simulink model "zumo_PID_controller_raw_values"  (R2014b)
settings: Solver=ode3  SolverMode=SingleTasking  StartTime=0.0  StopTime=4  FixedStep=0.01  RelTol=1e-3
InitFcn:
  | mapdata = processmap('mapTrackA.mat');
model workspace (MAT data in the model file):
  axleLength = Simulink.Parameter
  axleLength.Value = 9.8
  axleLength.Description = 'Distance between tire contact points
    | of the two wheels/treads
    | in units of centimeters.'
  axleLength.DataType = 'auto'
  commandPercmPerSecond = Simulink.Parameter
  commandPercmPerSecond.Value = 3.9547
  commandPercmPerSecond.Description = 'Convert units of ''command'' 
    | to units of ''cm/s''.
    | 
    | ''command'' is a value in the range [-256, 255].'
  commandPercmPerSecond.DataType = 'auto'
  symmetrizeMotors = Simulink.Parameter
  symmetrizeMotors.Value = 1
  symmetrizeMotors.Description = 'Scale one of the motor commands down 
    | (not up) to balance the motors. 
    | Once balanced, a value of x sent to either
    | motor will produce the same rate of rotation
    | in both motors.'
  symmetrizeMotors.DataType = 'auto'
  sampleTime = Simulink.Parameter
  sampleTime.Value = 0.01
  sampleTime.Description = 'Sample time (in seconds) of the trajectory simulator.'
  sampleTime.DataType = 'auto'
  commandThreshold = Simulink.Parameter
  commandThreshold.Value = 31.875
  commandThreshold.DataType = 'auto'
  lineThreshold = Simulink.Parameter
  lineThreshold.Value = 900
  lineThreshold.DataType = 'auto'
  velocity = Simulink.Parameter
  velocity.Value = 15
  velocity.Description = 'cm / s'
  velocity.DataType = 'auto'
  waveLength = Simulink.Parameter
  waveLength.Value = 8.6
  waveLength.Description = 'Units of cm.
    | 
    | The following condition must be satisfied: 
    | waveLength > 2*pi * velocity / sqrt(0.5 / sampleTime)
    | 
    | For reference,
    | robotLength = 8.6 cm
    | '
  waveLength.DataType = 'auto'
libraries: simulink x2, ZumoBotLib x2, arduinolib x1
settings Model: ExtModeTrigDuration=2  Creator=pkasseba  LastModifiedBy=sandip
settings OptimizationCC: OptimizeModelRefInitCode=on  LifeSpan=1
settings DebuggingCC: UnderspecifiedInitializationDetection=Classic  MergeDetectMultiDrivingBlocksExec=none  SolverPrmCheckMsg=none  StateNameClashWarn=warning
settings HardwareCC: ProdBitPerInt=16  ProdBitPerPointer=8  ProdIntDivRoundTo=Zero  ProdEndianess=LittleEndian  ProdWordSize=8  ProdHWDeviceType=Atmel->AVR
settings SFSimCC: SimParseCustomCode=off
settings RTWCC: SystemTargetFile=realtime.tlc  GenerateMakefile=off  TemplateMakefile=realtime.tmf  Description=Run on Target Hardware  RTWVerbose=off  ProcessScript=realtime_make_rtw_hook
settings STFCustomTargetCC: TargetLibSuffix=.a  GenerateSampleERTMain=on  ERTCustomFileBanners=on  SupportNonInlinedSFcns=off  SupportVariableSizeSignals=on  MATLABClassNameForMDSCustomization=Simulink.SoftwareTarget.ERTCustomization  GRTInterface=off  SystemTargetFile=realtime.tlc
settings ERTTargetCC: GenerateSampleERTMain=on  ParMdlRefBuildCompliant=off  CompOptLevelCompliant=off  ConcurrentExecutionCompliant=off  CombineOutputUpdateFcns=off  ERTFirstTimeCompliant=off  SupportContinuousTime=on  SupportVariableSizeSignals=on  ModelStepFunctionPrototypeControlCompliant=off  CPPClassGenCompliant=off  ExtModeTransport=3  ExtModeMexFile=ext_serial_win32_comm  ExtModeMexArgs=0 1 9600  InlinedParameterPlacement=NonHierarchical  ERTSrcFileBannerTemplate=realtime_code_template.cgt  ERTHdrFileBannerTemplate=realtime_code_template.cgt  ERTDataSrcFileTemplate=realtime_code_template.cgt  ERTDataHdrFileTemplate=realtime_code_template.cgt  ERTCustomFileTemplate=realtime_file_process.tlc

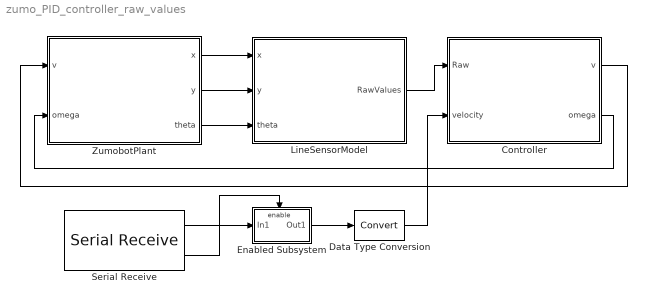
== system zumo_PID_controller_raw_values ==
  Controller : Subsystem
  Data Type Conversion : DataTypeConversion
  Enabled Subsystem : Subsystem  TreatAsAtomicUnit=on
  LineSensorModel : Subsystem  Variant=on
  Serial Receive : arduinolib/Serial Receive  portNumber=0  showOutStatus=on  sampleTime=0.02  blockPlatform=arduino
  ZumobotPlant : Subsystem  Variant=on
  wires:
  Controller/1(v) -> ZumobotPlant/1(v)
  ZumobotPlant/1(x) -> LineSensorModel/1(x)
  ZumobotPlant/2(y) -> LineSensorModel/2(y)
  LineSensorModel/1(RawValues) -> Controller/1(Raw)
  Controller/2(omega) -> ZumobotPlant/2(omega)
  ZumobotPlant/3(theta) -> LineSensorModel/3(theta)
  Serial Receive/1 -> Enabled Subsystem/1(In1)
  Serial Receive/2 -> Enabled Subsystem/Enable
  Enabled Subsystem/1(Out1) -> Data Type Conversion/1
  Data Type Conversion/1 -> Controller/2(velocity)

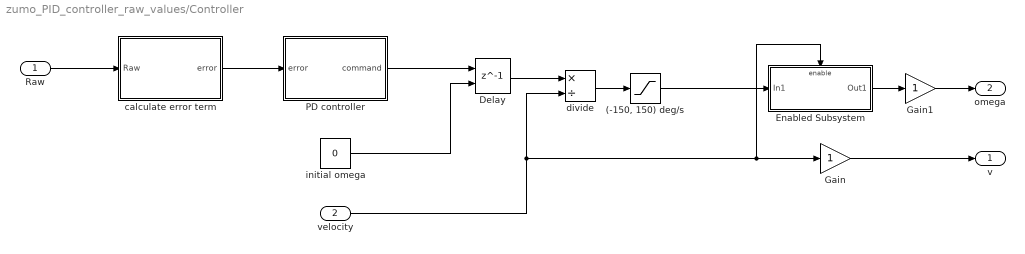
== system zumo_PID_controller_raw_values/Controller ==
  Raw : Inport
  velocity : Inport  Port=2
  "(-150, 150) deg/s" : Saturate  UpperLimit=150*pi/180  LowerLimit=-150*pi/180
  Delay : Delay  DelayLength=1  InitialConditionSource=Input port  InitialCondition=0
      settings: InputPortMap=u0,p4
  Enabled Subsystem : Subsystem  TreatAsAtomicUnit=on
  Gain : Gain
  Gain1 : Gain
  PD controller : Subsystem
  calculate error term : Subsystem
  divide : Product  Inputs=*/
  initial omega : Constant  Value=0
  v : Outport
  omega : Outport  Port=2
  wires:
  velocity/1 -> Gain/1, Enabled Subsystem/Enable, divide/2
  Delay/1 -> divide/1
  initial omega/1 -> Delay/2
  Raw/1 -> calculate error term/1(Raw)
  divide/1 -> "(-150, 150) deg/s"/1
  calculate error term/1(error) -> PD controller/1(error)
  PD controller/1(command) -> Delay/1
  "(-150, 150) deg/s"/1 -> Enabled Subsystem/1(In1)
  Enabled Subsystem/1(Out1) -> Gain1/1
  Gain/1 -> v/1
  Gain1/1 -> omega/1

== system zumo_PID_controller_raw_values/Enabled Subsystem ==
  In1 : Inport
  Enable : EnablePort
  Out1 : Outport  InitialOutput=0
  wires:
  In1/1 -> Out1/1

== system zumo_PID_controller_raw_values/LineSensorModel ==
  note: 1) Only subsystems can be added as variant choices at this level
      | 2) Blocks cannot be connected at this level as connectivity is
      | automatically determined at simulation, based on the active variant
  x : Inport
  y : Inport  Port=2
  theta : Inport  Port=3
  Simulation : Subsystem  VariantControl=sim==1
  Target : Subsystem  VariantControl=sim==0
  RawValues : Outport

== system zumo_PID_controller_raw_values/ZumobotPlant ==
  note: 1) Only subsystems can be added as variant choices at this level
      | 2) Blocks cannot be connected at this level as connectivity is
      | automatically determined at simulation, based on the active variant
  v : Inport
  omega : Inport  Port=2
  Simulation : Subsystem  VariantControl=sim==1
  Target : Subsystem  VariantControl=sim==0
  x : Outport
  y : Outport  Port=2
  theta : Outport  Port=3

== system zumo_PID_controller_raw_values/Controller/Enabled Subsystem ==
  In1 : Inport
  Enable : EnablePort
  Out1 : Outport  OutputWhenDisabled=reset  InitialOutput=0
  wires:
  In1/1 -> Out1/1

== system zumo_PID_controller_raw_values/Controller/PD controller ==
  error : Inport
  2*alpha : Gain  Gain=2*(2*pi*velocity/waveLength)
  Discrete Derivative : simulink/Discrete/Discrete Derivative  gainval=1.0  ICPrevScaledInput=0.0  InputProcessing=Inherited  OutMin=[]  OutMax=[]  OutDataType=fixdt(1, 16)  OutScaling=2^-10  DoSatur=off
  Sum : Sum  Inputs=|++
  alpha^2 : Gain  Gain=(2*pi*velocity/waveLength)^2
  zeta : Gain  Gain=0.4
  command : Outport
  wires:
  zeta/1 -> 2*alpha/1
  2*alpha/1 -> Discrete Derivative/1
  alpha^2/1 -> Sum/1
  Sum/1 -> command/1
  Discrete Derivative/1 -> Sum/2
  error/1 -> alpha^2/1, zeta/1

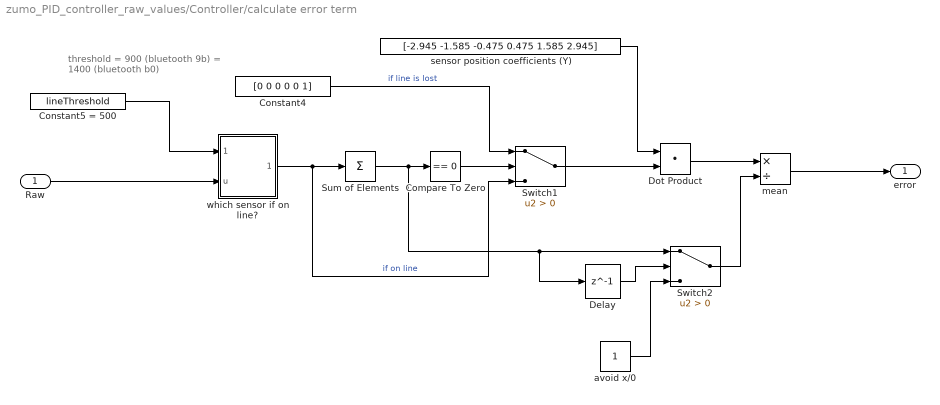
== system zumo_PID_controller_raw_values/Controller/calculate error term ==
  note: threshold = 900 (bluetooth 9b)
      | = 1400 (bluetooth b0)
  Raw : Inport
  Compare To Zero : simulink/Logic and Bit Operations/Compare To Zero  relop===  OutDataTypeStr=boolean
  Constant4 : Constant  Value=[0 0 0 0 0 1]
  Constant5 = 500 : Constant  Value=lineThreshold
  Delay : Delay  DelayLength=1  InitialCondition=0
  Dot Product : DotProduct  InputSameDT=on  OutDataTypeStr=Inherit: Inherit via internal rule
  Sum of Elements : Sum  Inputs=+
  Switch1 : Switch  Criteria=u2 > Threshold
  Switch2 : Switch  Criteria=u2 > Threshold
  avoid x/0 : Constant
  mean : Product  Inputs=*/
  sensor position coefficients (Y) : Constant  Value=[-2.945 -1.585 -0.475 0.475 1.585 2.945]
  which sensor if on line? : Subsystem
  error : Outport
  wires:
  Constant4/1 -> Switch1/1  "if line is lost"
  Constant5 = 500/1 -> which sensor if on line?/1(threshold)
  Dot Product/1 -> mean/1
  sensor position coefficients (Y)/1 -> Dot Product/1
  Raw/1 -> which sensor if on line?/2(u)
  which sensor if on line?/1(Out1) -> Switch1/3, Sum of Elements/1  "if on line"
  Switch2/1 -> mean/2
  avoid x/0/1 -> Switch2/3
  Switch1/1 -> Dot Product/2
  mean/1 -> error/1
  Compare To Zero/1 -> Switch1/2
  Sum of Elements/1 -> Delay/1, Switch2/1, Compare To Zero/1
  Delay/1 -> Switch2/2

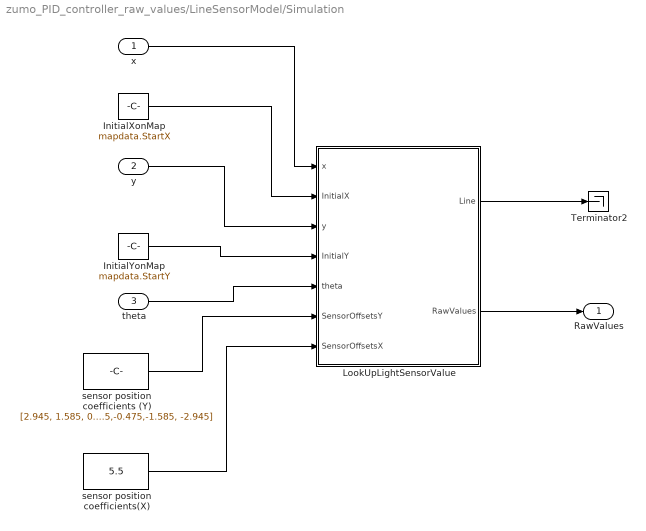
== system zumo_PID_controller_raw_values/LineSensorModel/Simulation ==
  x : Inport
  y : Inport  Port=2
  theta : Inport  Port=3
  InitialXonMap : Constant  Value=mapdata.StartX
  InitialYonMap : Constant  Value=mapdata.StartY
  LookUpLightSensorValue : Subsystem
  Terminator2 : Terminator
  sensor position coefficients (Y) : Constant  Value=[2.945, 1.585, 0.475,-0.475,-1.585, -2.945]
  sensor position coefficients(X) : Constant  Value=5.5
  RawValues : Outport
  wires:
  LookUpLightSensorValue/1(Line) -> Terminator2/1
  LookUpLightSensorValue/2(RawValues) -> RawValues/1
  InitialYonMap/1 -> LookUpLightSensorValue/4(InitialY)
  theta/1 -> LookUpLightSensorValue/5(theta)
  sensor position coefficients (Y)/1 -> LookUpLightSensorValue/6(SensorOffsetsY)
  y/1 -> LookUpLightSensorValue/3(y)
  InitialXonMap/1 -> LookUpLightSensorValue/2(InitialX)
  x/1 -> LookUpLightSensorValue/1(x)
  sensor position coefficients(X)/1 -> LookUpLightSensorValue/7(SensorOffsetsX)

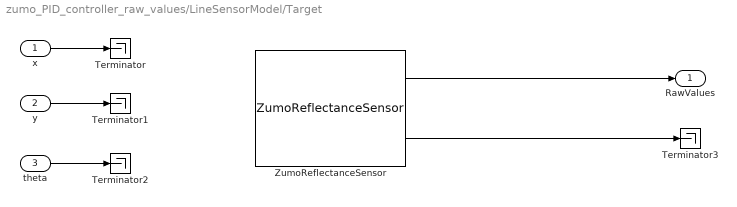
== system zumo_PID_controller_raw_values/LineSensorModel/Target ==
  x : Inport
  y : Inport  Port=2
  theta : Inport  Port=3
  Terminator{,1..3} (4 alike) : Terminator
  ZumoReflectanceSensor : ZumoBotLib/ZumoReflectanceSensor  sampleTime_dd=0.02  emitterPin_dd=255  debug_dd=off
  RawValues : Outport
  wires:
  ZumoReflectanceSensor/1 -> RawValues/1
  ZumoReflectanceSensor/2 -> Terminator3/1
  x/1 -> Terminator/1
  y/1 -> Terminator1/1
  theta/1 -> Terminator2/1

== system zumo_PID_controller_raw_values/ZumobotPlant/Simulation ==
  v : Inport
  omega : Inport  Port=2
  motor command conversion : Subsystem
  simulated trajectory : Subsystem
  x : Outport
  y : Outport  Port=2
  theta : Outport  Port=3
  wires:
  v/1 -> motor command conversion/1(v)
  simulated trajectory/1(x) -> x/1
  simulated trajectory/2(y) -> y/1
  motor command conversion/1(v_L v_R) -> simulated trajectory/1(v_L v_R)
  omega/1 -> motor command conversion/2(omega)
  simulated trajectory/3(theta) -> theta/1

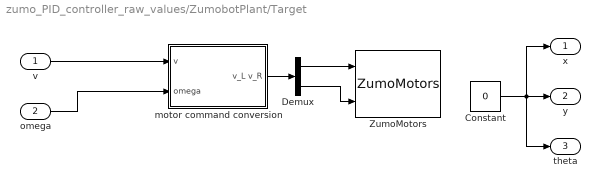
== system zumo_PID_controller_raw_values/ZumobotPlant/Target ==
  v : Inport
  omega : Inport  Port=2
  Constant : Constant  Value=0
  Demux : Demux  Outputs=2
  ZumoMotors : ZumoBotLib/ZumoMotors  flipLeft=off  flipRight=off
  motor command conversion : Subsystem
  x : Outport
  y : Outport  Port=2
  theta : Outport  Port=3
  wires:
  motor command conversion/1(v_L v_R) -> Demux/1
  Demux/1 -> ZumoMotors/1
  Demux/2 -> ZumoMotors/2
  v/1 -> motor command conversion/1(v)
  omega/1 -> motor command conversion/2(omega)
  Constant/1 -> theta/1, x/1, y/1

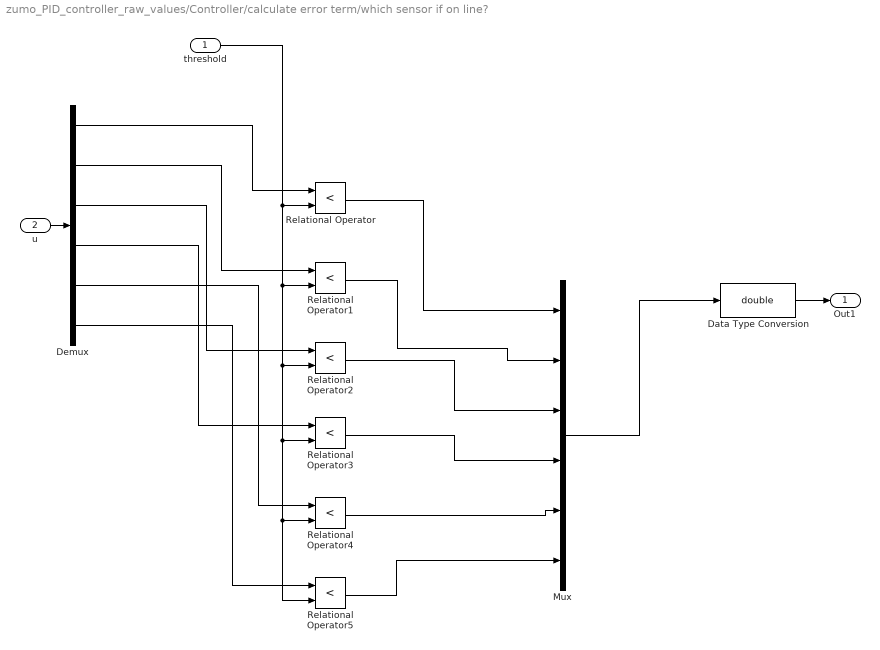
== system zumo_PID_controller_raw_values/Controller/calculate error term/which sensor if on line? ==
  threshold : Inport
  u : Inport  Port=2
  Data Type Conversion : DataTypeConversion  OutDataTypeStr=double
  Demux : Demux  Outputs=6
  Mux : Mux  Inputs=6
  Relational Operator{,1..5} (6 alike) : RelationalOperator  Operator=<  OutDataTypeStr=boolean
  Out1 : Outport
  wires:
  Mux/1 -> Data Type Conversion/1
  u/1 -> Demux/1
  Demux/1 -> Relational Operator/1
  Demux/2 -> Relational Operator1/1
  Demux/3 -> Relational Operator2/1
  Demux/4 -> Relational Operator3/1
  Demux/5 -> Relational Operator4/1
  Demux/6 -> Relational Operator5/1
  threshold/1 -> Relational Operator5/2, Relational Operator4/2, Relational Operator3/2, Relational Operator2/2, Relational Operator1/2, Relational Operator/2
  Relational Operator1/1 -> Mux/2
  Relational Operator2/1 -> Mux/3
  Relational Operator/1 -> Mux/1
  Relational Operator3/1 -> Mux/4
  Relational Operator5/1 -> Mux/6
  Data Type Conversion/1 -> Out1/1
  Relational Operator4/1 -> Mux/5

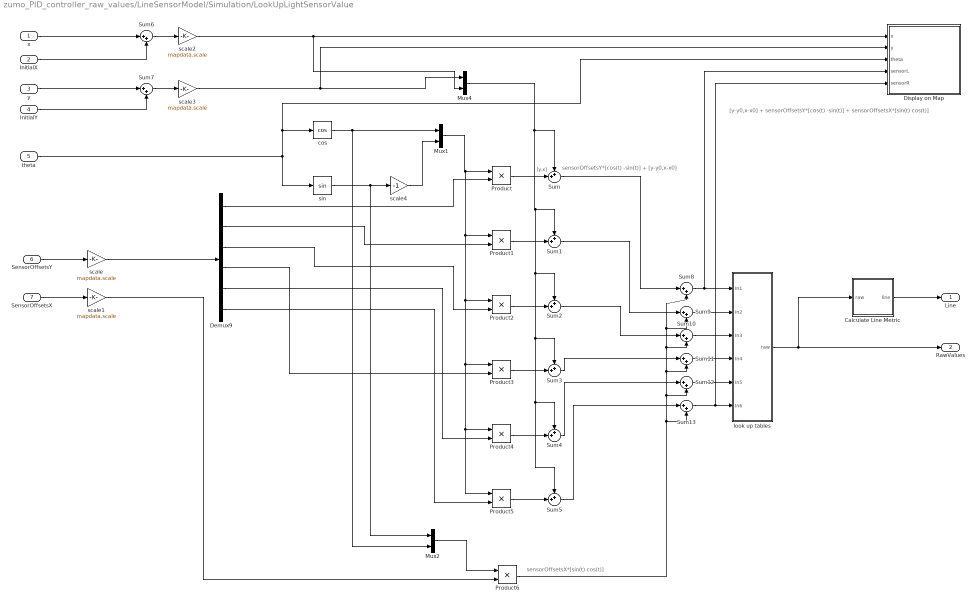
== system zumo_PID_controller_raw_values/LineSensorModel/Simulation/LookUpLightSensorValue ==
  note: [y-y0,x-x0] + sensorOffsetsY*[cos(t) -sin(t)] + sensorOffsetsX*[sin(t) cos(t)]
  note: sensorOffsetsY*[cos(t) -sin(t)] + [y-y0,x-x0]
  note: sensorOffsetsX*[sin(t) cos(t)]
  x : Inport
  InitialX : Inport  Port=2
  y : Inport  Port=3
  InitialY : Inport  Port=4
  theta : Inport  Port=5
  SensorOffsetsY : Inport  Port=6
  SensorOffsetsX : Inport  Port=7
  Calculate Line Metric : Subsystem
  Demux9 : Demux  Outputs=6
  Display on Map : MATLAB Function  TreatAsAtomicUnit=on
  Mux1 : Mux  Inputs=2
  Mux2 : Mux  Inputs=2
  Mux4 : Mux  Inputs=2
  Product{,1..6} (7 alike) : Product
  Sum{,1..5} (6 alike) : Sum  Inputs=++|
  Sum{6..13} (8 alike) : Sum  Inputs=|++
  cos : Trigonometry  Operator=cos
  look up tables : Subsystem
  scale{,1..3} (4 alike) : Gain  Gain=mapdata.scale
  scale4 : Gain  Gain=-1
  sin : Trigonometry
  Line : Outport
  RawValues : Outport  Port=2
  wires:
  SensorOffsetsY/1 -> scale/1
  Mux1/1 -> Product5/1, Product4/1, Product3/1, Product2/1, Product1/1, Product/1
  Product/1 -> Sum/2
  Product1/1 -> Sum1/2
  Product2/1 -> Sum2/2
  Product4/1 -> Sum4/2
  Product3/1 -> Sum3/2
  Product5/1 -> Sum5/2
  Sum/1 -> Sum8/1
  Sum5/1 -> Sum13/1
  scale/1 -> Demux9/1
  Demux9/4 -> Product3/2
  Demux9/5 -> Product4/2
  Demux9/3 -> Product2/2
  Demux9/6 -> Product5/2
  Demux9/2 -> Product1/2
  Demux9/1 -> Product/2
  Mux4/1 -> Sum/1, Sum5/1, Sum4/1, Sum3/1, Sum2/1, Sum1/1  "[y,x]"
  SensorOffsetsX/1 -> scale1/1
  scale1/1 -> Product6/2
  Mux2/1 -> Product6/1
  Product6/1 -> Sum13/2, Sum12/2, Sum11/2, Sum10/2, Sum9/2, Sum8/2
  x/1 -> Sum6/1
  Sum6/1 -> scale2/1
  InitialX/1 -> Sum6/2
  y/1 -> Sum7/1
  Sum7/1 -> scale3/1
  InitialY/1 -> Sum7/2
  scale2/1 -> Mux4/2, Display on Map/1(x)
  scale3/1 -> Mux4/1, Display on Map/2(y)
  Calculate Line Metric/1(line) -> Line/1
  look up tables/1(raw) -> Calculate Line Metric/1(raw), RawValues/1
  Sum1/1 -> Sum9/1
  Sum2/1 -> Sum10/1
  Sum3/1 -> Sum11/1
  Sum4/1 -> Sum12/1
  Sum8/1 -> Display on Map/4(sensorL), look up tables/1(In1)
  Sum9/1 -> look up tables/2(In2)
  Sum10/1 -> look up tables/3(In3)
  Sum11/1 -> look up tables/4(In4)
  Sum12/1 -> look up tables/5(In5)
  Sum13/1 -> Display on Map/5(sensorR), look up tables/6(In6)
  sin/1 -> Mux2/1, scale4/1
  cos/1 -> Mux2/2, Mux1/1
  theta/1 -> Display on Map/3(theta), cos/1, sin/1
  scale4/1 -> Mux1/2

== system zumo_PID_controller_raw_values/ZumobotPlant/Simulation/motor command conversion ==
  note: or in matrix notation,
  note: v_L  = v - omega * axleLength/2
      | v_R = v + omega * axleLength/2
  note: [v_L; v_R] = [1 -axleLength/2; 1 axleLength/2] * [v; omega]
  v : Inport
  omega : Inport  Port=2
  Mux : Mux  Inputs=2
  Saturation [-256 255] : Saturate  UpperLimit=255  LowerLimit=-256
  change parameters : Gain  Gain=[1 -axleLength/2; 1 axleLength/2]  Multiplication=Matrix(K*u)
  change units : Gain  Gain=commandPercmPerSecond
  symmetrize motors : Gain  Gain=[1 symmetrizeMotors]
  v_L v_R : Outport
  wires:
  change parameters/1 -> symmetrize motors/1  "v_L v_R"
  change units/1 -> Saturation [-256 255]/1  "v_L v_R (command)"
  symmetrize motors/1 -> change units/1  "v_L v_R (cm/s)"
  Saturation [-256 255]/1 -> v_L v_R/1
  Mux/1 -> change parameters/1
  omega/1 -> Mux/2
  v/1 -> Mux/1

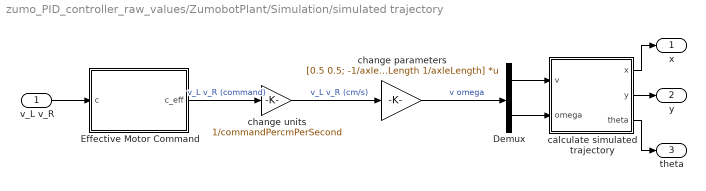
== system zumo_PID_controller_raw_values/ZumobotPlant/Simulation/simulated trajectory ==
  v_L v_R : Inport
  Demux : Demux  Outputs=2
  Effective Motor Command : Subsystem
  calculate simulated trajectory : Subsystem
  change parameters : Gain  Gain=[0.5 0.5; -1/axleLength 1/axleLength]  Multiplication=Matrix(K*u)
  change units : Gain  Gain=1/commandPercmPerSecond
  x : Outport
  y : Outport  Port=2
  theta : Outport  Port=3
  wires:
  Demux/2 -> calculate simulated trajectory/2(omega)
  Demux/1 -> calculate simulated trajectory/1(v)
  v_L v_R/1 -> Effective Motor Command/1(c)
  Effective Motor Command/1(c_eff) -> change units/1  "v_L v_R (command)"
  change units/1 -> change parameters/1  "v_L v_R (cm/s)"
  change parameters/1 -> Demux/1  "v omega"
  calculate simulated trajectory/2(y) -> y/1
  calculate simulated trajectory/1(x) -> x/1
  calculate simulated trajectory/3(theta) -> theta/1

== system zumo_PID_controller_raw_values/ZumobotPlant/Target/motor command conversion ==
  note: or in matrix notation,
  note: v_L  = v - omega * axleLength/2
      | v_R = v + omega * axleLength/2
  note: [v_L; v_R] = [1 -axleLength/2; 1 axleLength/2] * [v; omega]
  v : Inport
  omega : Inport  Port=2
  Gain : Gain
  Mux : Mux  Inputs=2
  Saturation [-256 255] : Saturate  UpperLimit=255  LowerLimit=-256
  change parameters : Gain  Gain=[1 -axleLength/2; 1 axleLength/2]  Multiplication=Matrix(K*u)
  change units : Gain  Gain=commandPercmPerSecond
  symmetrize motors : Gain  Gain=[1 symmetrizeMotors]
  v_L v_R : Outport
  wires:
  change parameters/1 -> symmetrize motors/1  "v_L v_R"
  change units/1 -> Saturation [-256 255]/1  "v_L v_R (command)"
  symmetrize motors/1 -> change units/1  "v_L v_R (cm/s)"
  Saturation [-256 255]/1 -> Gain/1
  Mux/1 -> change parameters/1
  omega/1 -> Mux/2
  v/1 -> Mux/1
  Gain/1 -> v_L v_R/1

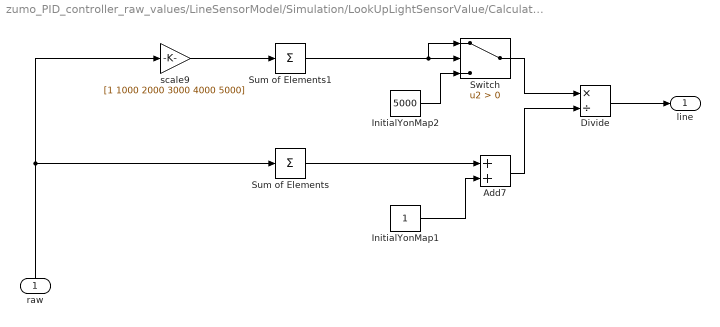
== system zumo_PID_controller_raw_values/LineSensorModel/Simulation/LookUpLightSensorValue/Calculate Line Metric ==
  raw : Inport
  Add7 : Sum
  Divide : Product  Inputs=*/
  InitialYonMap1 : Constant
  InitialYonMap2 : Constant  Value=5000
  Sum of Elements : Sum  Inputs=+
  Sum of Elements1 : Sum  Inputs=+
  Switch : Switch  Criteria=u2 > Threshold
  scale9 : Gain  Gain=[1 1000 2000 3000 4000 5000]
  line : Outport
  wires:
  Sum of Elements/1 -> Add7/1
  Divide/1 -> line/1
  InitialYonMap1/1 -> Add7/2
  Add7/1 -> Divide/2
  Sum of Elements1/1 -> Switch/1, Switch/2
  Switch/1 -> Divide/1
  InitialYonMap2/1 -> Switch/3
  scale9/1 -> Sum of Elements1/1
  raw/1 -> scale9/1, Sum of Elements/1

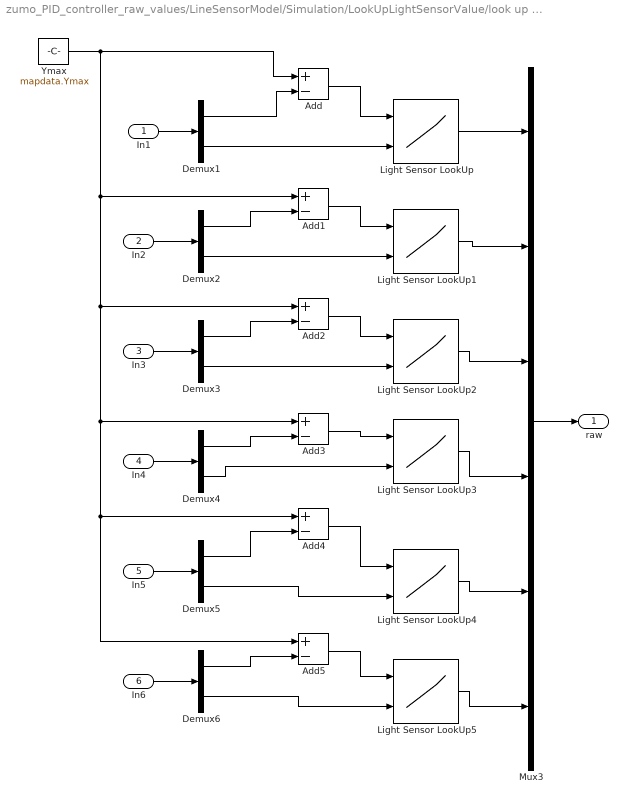
== system zumo_PID_controller_raw_values/LineSensorModel/Simulation/LookUpLightSensorValue/look up tables ==
  In1 : Inport
  In2 : Inport  Port=2
  In3 : Inport  Port=3
  In4 : Inport  Port=4
  In5 : Inport  Port=5
  In6 : Inport  Port=6
  Add{,1..5} (6 alike) : Sum  Inputs=+-
  Demux{1..6} (6 alike) : Demux  Outputs=2
  Light Sensor LookUp{,1..5} (6 alike) : Lookup_n-D  BreakpointsForDimension1=mapdata.yBreakPoints  BreakpointsForDimension2=mapdata.xBreakPoints  Table=mapdata.ReflectanceData  InterpMethod=Flat  ExtrapMethod=Clip  UseLastTableValue=on  RndMeth=Round  SaturateOnIntegerOverflow=on  InputSameDT=on
  Mux3 : Mux  Inputs=6
  Ymax : Constant  Value=mapdata.Ymax
  raw : Outport
  wires:
  Demux1/1 -> Add/2
  Demux1/2 -> Light Sensor LookUp/2
  Demux2/2 -> Light Sensor LookUp1/2
  In2/1 -> Demux2/1
  Demux3/2 -> Light Sensor LookUp2/2
  Demux4/2 -> Light Sensor LookUp3/2
  Demux5/2 -> Light Sensor LookUp4/2
  Demux6/2 -> Light Sensor LookUp5/2
  In3/1 -> Demux3/1
  In4/1 -> Demux4/1
  In5/1 -> Demux5/1
  Light Sensor LookUp4/1 -> Mux3/5
  Light Sensor LookUp1/1 -> Mux3/2
  Light Sensor LookUp5/1 -> Mux3/6
  Light Sensor LookUp3/1 -> Mux3/4
  Light Sensor LookUp2/1 -> Mux3/3
  Light Sensor LookUp/1 -> Mux3/1
  Mux3/1 -> raw/1
  Add/1 -> Light Sensor LookUp/1
  Demux2/1 -> Add1/2
  Add1/1 -> Light Sensor LookUp1/1
  Demux3/1 -> Add2/2
  Add2/1 -> Light Sensor LookUp2/1
  Demux4/1 -> Add3/2
  Add3/1 -> Light Sensor LookUp3/1
  Demux5/1 -> Add4/2
  Add4/1 -> Light Sensor LookUp4/1
  Demux6/1 -> Add5/2
  Ymax/1 -> Add5/1, Add4/1, Add3/1, Add2/1, Add1/1, Add/1
  Add5/1 -> Light Sensor LookUp5/1
  In6/1 -> Demux6/1
  In1/1 -> Demux1/1

== system zumo_PID_controller_raw_values/ZumobotPlant/Simulation/simulated trajectory/Effective Motor Command ==
  note: Zumobot does not move when given a command
      | with an abs less than 50 on a smooth surface,
      | so such commands are effectively 0.
  note: Do not saturate this signal.The process of symmetrizing
      | the motor commands gives rise to this artificial signal,
      | which can exceed the value of 255.
  c : Inport
  Abs : Abs
  Constant1 : Constant  Value=0
  Sum : Sum  Inputs=|+-
  Switch : Switch
  command threshold : Constant  Value=commandThreshold
  symmetrize motors : Gain  Gain=[1 1/symmetrizeMotors]
  c_eff : Outport
  wires:
  Switch/1 -> c_eff/1
  symmetrize motors/1 -> Abs/1, Switch/1
  Sum/1 -> Switch/2
  Abs/1 -> Sum/1
  command threshold/1 -> Sum/2
  c/1 -> symmetrize motors/1  "v_L v_R"
  Constant1/1 -> Switch/3

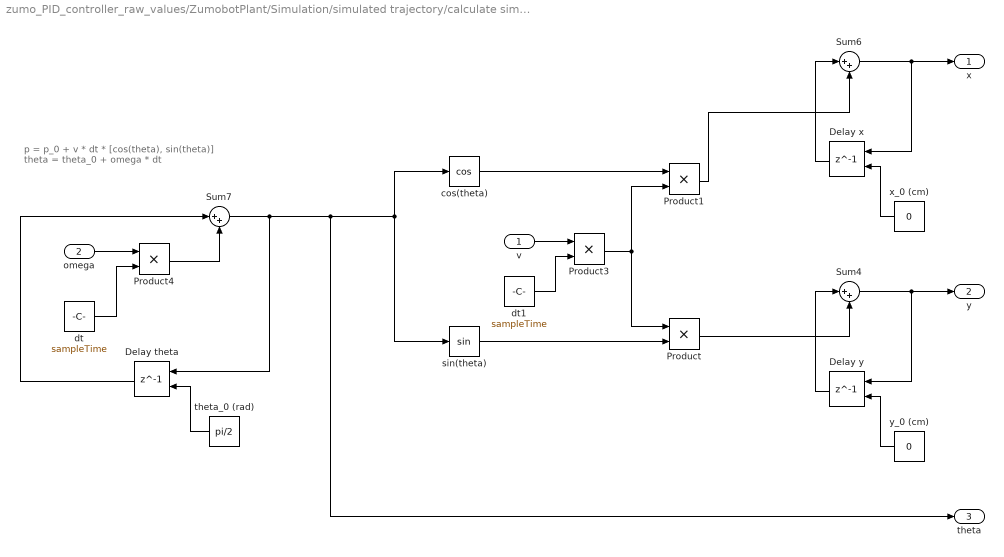
== system zumo_PID_controller_raw_values/ZumobotPlant/Simulation/simulated trajectory/calculate simulated trajectory ==
  note: p = p_0 + v * dt * [cos(theta), sin(theta)]
      | theta = theta_0 + omega * dt
  v : Inport
  omega : Inport  Port=2
  Delay theta : Delay  DelayLength=1  InitialConditionSource=Input port  InitialCondition=0  SampleTime=sampleTime
      settings: InputPortMap=u0,p4
  Delay x : Delay  DelayLength=1  InitialConditionSource=Input port  InitialCondition=0
      settings: InputPortMap=u0,p4
  Delay y : Delay  DelayLength=1  InitialConditionSource=Input port  InitialCondition=0
      settings: InputPortMap=u0,p4
  Product{,1,3..4} (4 alike) : Product
  Sum4 : Sum  Inputs=|++
  Sum6 : Sum  Inputs=|++
  Sum7 : Sum  Inputs=|++
  cos(theta) : Trigonometry  Operator=cos
  dt : Constant  Value=sampleTime
  dt1 : Constant  Value=sampleTime
  sin(theta) : Trigonometry
  theta_0 (rad) : Constant  Value=pi/2
  x_0 (cm) : Constant  Value=0
  y_0 (cm) : Constant  Value=0
  x : Outport
  y : Outport  Port=2
  theta : Outport  Port=3
  wires:
  dt/1 -> Product4/2
  omega/1 -> Product4/1
  Product4/1 -> Sum7/2
  Product3/1 -> Product/1, Product1/2
  v/1 -> Product3/1
  dt1/1 -> Product3/2
  Product1/1 -> Sum6/2
  Delay x/1 -> Sum6/1
  Sum6/1 -> Delay x/1, x/1
  Product/1 -> Sum4/2
  Delay y/1 -> Sum4/1
  sin(theta)/1 -> Product/2
  cos(theta)/1 -> Product1/1
  Sum4/1 -> y/1, Delay y/1
  Delay theta/1 -> Sum7/1
  Sum7/1 -> theta/1, cos(theta)/1, sin(theta)/1, Delay theta/1
  theta_0 (rad)/1 -> Delay theta/2
  y_0 (cm)/1 -> Delay y/2
  x_0 (cm)/1 -> Delay x/2

== matlab function zumo_PID_controller_raw_values/LineSensorModel/Simulation/LookUpLightSensorValue/Display on Map ==
  data: x input; y input; theta input; sensorL input; sensorR input
function fcn(x,y, theta, sensorL,sensorR)
%#codegen

coder.extrinsic('dispOnMap');
dispOnMap(x,y, theta, sensorL, sensorR);
